simulink model "Two_IBR_Impulse"  (R2022b)
settings: Solver=FixedStepAuto  StartTime=0  StopTime=6  FixedStep=Ts  RelTol=1e-3
undefined symbols (not defined in the file or in its folder): ApparatusDiscreDamping, ApparatusPara, ApparatusPowerFlow, ApparatusType, OtherInputs, R, Ts, Wbase, x_e, Ybase, Zbase
libraries: spsGroundLib x12, SimplusGT x12, spsThreePhaseParallelRLCBranchLib x8, spsThreePhaseBreakerLib x5, spsThreePhaseSeriesRLCBranchLib x3, spspowerguiLib x1
settings Model: Creator=yz34218  LastModifiedBy=yz34218

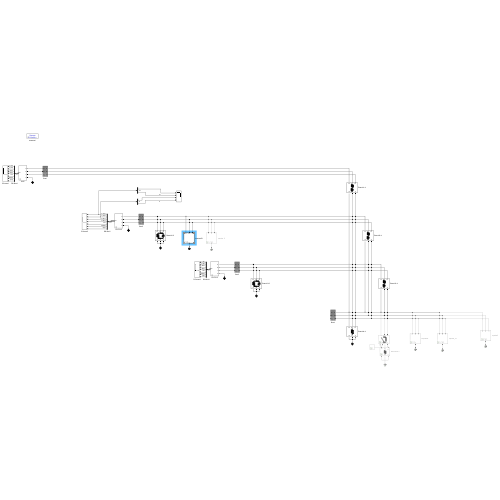
[thumbnail: Simulink's stored preview of the top-level diagram]
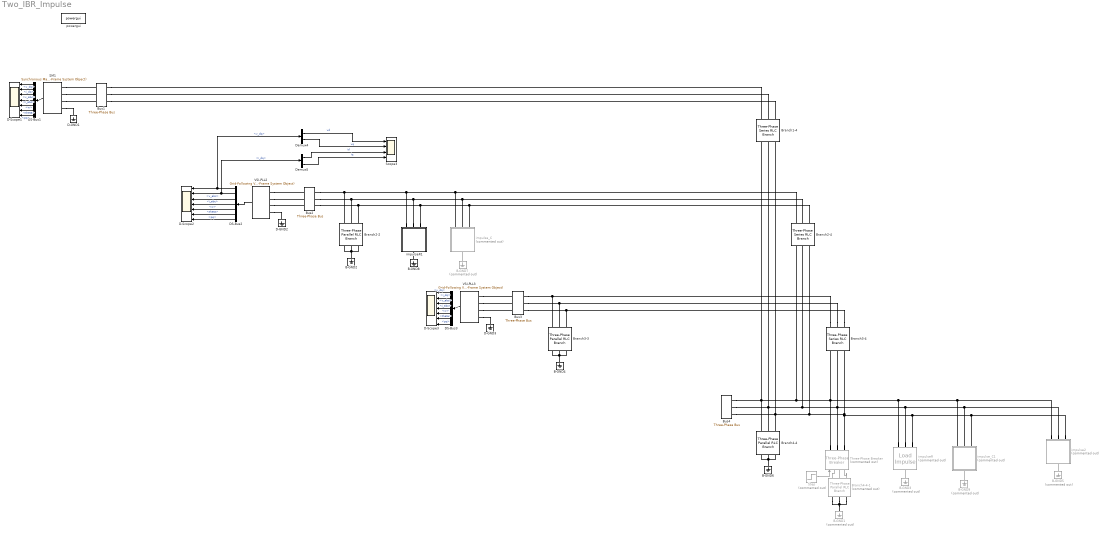
== system Two_IBR_Impulse ==
  B-GND{1,3,5,7,9} (5 alike) : spsGroundLib/Ground  Commented=on  LConnTagsString=a
  B-GND{2,4,6,8} (4 alike) : spsGroundLib/Ground  LConnTagsString=a
  Branch1-4 : spsThreePhaseSeriesRLCBranchLib/Three-Phase Series RLC Branch  LConnTagsString=A|B|C  RConnTagsString=A|B|C  BranchType=RL  Resistance=(0.01)*Zbase  Inductance=(0.1)*Zbase/Wbase  Capacitance=1e-6  Measurements=None
  Branch2-2 : spsThreePhaseParallelRLCBranchLib/Three-Phase Parallel RLC Branch  LConnTagsString=A|B|C  RConnTagsString=A|B|C  BranchType=RC  Resistance=(13.8626)*Zbase  Inductance=(Inf)*Zbase/Wbase  Capacitance=(0.3)*Ybase/Wbase  Measurements=None
  Branch2-4 : spsThreePhaseSeriesRLCBranchLib/Three-Phase Series RLC Branch  LConnTagsString=A|B|C  RConnTagsString=A|B|C  BranchType=RL  Resistance=(0.03)*Zbase  Inductance=(0.3)*Zbase/Wbase  Capacitance=1e-6  Measurements=None
  Branch3-3 : spsThreePhaseParallelRLCBranchLib/Three-Phase Parallel RLC Branch  LConnTagsString=A|B|C  RConnTagsString=A|B|C  BranchType=RC  Resistance=(13.8626)*Zbase  Inductance=(Inf)*Zbase/Wbase  Capacitance=(0.3)*Ybase/Wbase  Measurements=None
  Branch3-4 : spsThreePhaseSeriesRLCBranchLib/Three-Phase Series RLC Branch  LConnTagsString=A|B|C  RConnTagsString=A|B|C  BranchType=RL  Resistance=(0.03)*Zbase  Inductance=(0.3)*Zbase/Wbase  Capacitance=1e-6  Measurements=None
  Branch4-4 : spsThreePhaseParallelRLCBranchLib/Three-Phase Parallel RLC Branch  LConnTagsString=A|B|C  RConnTagsString=A|B|C  BranchType=R  Resistance=(11.3805)*Zbase  Inductance=(Inf)*Zbase/Wbase  Capacitance=(0)*Ybase/Wbase  Measurements=None
  Branch4-4-1 : spsThreePhaseParallelRLCBranchLib/Three-Phase Parallel RLC Branch  Commented=on  LConnTagsString=A|B|C  RConnTagsString=A|B|C  BranchType=R  Resistance=(11.3805)*Zbase*4  Inductance=(Inf)*Zbase/Wbase  Capacitance=(0)*Ybase/Wbase  Measurements=None
  Bus{1..4} (4 alike) : SimplusGT/Three-Phase Bus  Vbase=1  Sbase=1
      settings: SourceProductName=Simplus Grid Tool
  D-GND1 : spsGroundLib/Ground  LConnTagsString=a
  D-GND2 : spsGroundLib/Ground  LConnTagsString=a
  D-GND3 : spsGroundLib/Ground  LConnTagsString=a
  D-Scope1 : Scope  NumInputPorts=7
  D-Scope2 : Scope  NumInputPorts=7
  D-Scope3 : Scope  NumInputPorts=7
  DS-Bus1 : BusSelector  OutputSignals=v_dq,i_dq,v_abc,i_abc,w,theta,pq
  DS-Bus2 : BusSelector  OutputSignals=v_dq,i_dq,v_abc,i_abc,w,theta,pq
  DS-Bus3 : BusSelector  OutputSignals=v_dq,i_dq,v_abc,i_abc,w,theta,pq
  Demux4 : Demux  Outputs=2
  Demux5 : Demux  Outputs=2
  SM1 : SimplusGT/Synchronous Machine (dq-Frame System Object)  Ts=Ts  Sbase=Sbase  Vbase=Vbase  Wbase=Wbase  ApparatusType=ApparatusType{1}  ApparatusPara=ApparatusPara{1}  PowerFlow=ApparatusPowerFlow{1}  x0=x_e{1}  OtherInputs=OtherInputs{1}  DiscreMethod=Hybrid Trapezoidal  EnableInsideModification=off  DiscreDampingFlag=on  DiscreDampingValue=ApparatusDiscreDamping{1}  LinearizationTimes=1  DirectFeedthrough=off
      settings: SourceProductName=Simplus Grid Tool
  Scope3 : Scope  NumInputPorts=4
  Step : Step  Commented=on  Time=3  SampleTime=0
  Three-Phase Breaker : spsThreePhaseBreakerLib/Three-Phase Breaker  Commented=on  InitialState=open  SwitchA=on  SwitchB=on  SwitchC=on  SwitchTimes="[1/60  5/60]"  External=on  BreakerResistance=0.01  SnubberResistance=1e6  SnubberCapacitance=inf  Measurements=None
  VSI-PLL2 : SimplusGT/Grid-Following Voltage-Source Inverter (dq-Frame System Object)  Ts=Ts  Sbase=Sbase  Vbase=Vbase  Wbase=Wbase  ApparatusType=ApparatusType{2}  ApparatusPara=ApparatusPara{2}  PowerFlow=ApparatusPowerFlow{2}  x0=x_e{2}  OtherInputs=OtherInputs{2}  DiscreMethod=Hybrid Trapezoidal  EnableInsideModification=off  DiscreDampingFlag=on  DiscreDampingValue=ApparatusDiscreDamping{2}  LinearizationTimes=1  DirectFeedthrough=off
      settings: SourceProductName=Simplus Grid Tool
  VSI-PLL3 : SimplusGT/Grid-Following Voltage-Source Inverter (dq-Frame System Object)  Ts=Ts  Sbase=Sbase  Vbase=Vbase  Wbase=Wbase  ApparatusType=ApparatusType{3}  ApparatusPara=ApparatusPara{3}  PowerFlow=ApparatusPowerFlow{3}  x0=x_e{3}  OtherInputs=OtherInputs{3}  DiscreMethod=Hybrid Trapezoidal  EnableInsideModification=off  DiscreDampingFlag=on  DiscreDampingValue=ApparatusDiscreDamping{3}  LinearizationTimes=1  DirectFeedthrough=off
      settings: SourceProductName=Simplus Grid Tool
  impulse2 : Subsystem  Commented=on  AncestorBlock=SimplusGT/Load Impulse  mask{t0=6, dt=0.01, C=(11.3805)*Zbase*0.2}
      settings: LibrarySourceBlock=SimplusGT/Load Impulse
  impulseR : SimplusGT/Load Impulse  Commented=on  t0=3  dt=0.01  R=(11.3805)*Zbase*5
      settings: SourceProductName=Simplus Grid Tool
  impulseR1 : Subsystem  AncestorBlock=SimplusGT/Load Impulse  mask{t0=3, dt=0.01, R=(13.8626)*Zbase*2}
      settings: LibrarySourceBlock=SimplusGT/Load Impulse
  impulse_C : Subsystem  Commented=on  AncestorBlock=SimplusGT/Load Impulse  mask{t0=5, dt=0.01, C=(0.3)*Ybase/Wbase*0.1}
      settings: LibrarySourceBlock=SimplusGT/Load Impulse
  impulse_C1 : Subsystem  Commented=on  AncestorBlock=SimplusGT/Load Impulse  mask{t0=6, dt=0.01, C=(0.3)*Ybase/Wbase*0.1}
      settings: LibrarySourceBlock=SimplusGT/Load Impulse
  powergui : spspowerguiLib/powergui  Priority=1  SimulationMode=Discrete  SampleTime=Ts  frequency=60  Iterations=50  frequencyindice=0  Pbase=100e6  ErrMax=1e-4  UnitsV=kV  UnitsW=MW  buscounter=0  FunctionMessages=off  echomessages=off  EnableUseOfTLC=off  CurrentSourceSwitches=off  DisableSnubberDevices=off  DisableRonSwitches=off  DisableVfSwitches=off  DisplayEquations=off  AutomaticDiscreteSolvers=off  SolverType=Tustin/Backward Euler (TBE)  Interpol=off  ExternalGateDelay=off  methode=off  Ts=100  x0status=blocks  SPID=on  SwTol=0  HookPort=off  NonlinearTolerance=1e-4  nMaxIteration=100  ContinueOnMaxIteration=off  RestoreLinks=warning  ResistiveCurrentMeasurement=off  Frange=[0:2:500]  Ylog=off  Xlog=on  ShowGrid=off  save=off  variable=ZData  structure=0  ZoomFFT=off  StartTime=0.0  cycles=1  DisplayStyle=1  fundamental=60  FreqAxis=off  MaxFrequency=1000  frequencyindicesteady=1  RmsSteady=1  display=off
  wires:
  SM1/1 -> DS-Bus1/1
  DS-Bus1/1 -> D-Scope1/1  "<v_dq>"
  DS-Bus1/2 -> D-Scope1/2  "<i_dq>"
  DS-Bus1/3 -> D-Scope1/3  "<v_abc>"
  DS-Bus1/4 -> D-Scope1/4  "<i_abc>"
  DS-Bus1/5 -> D-Scope1/5  "<w>"
  DS-Bus1/6 -> D-Scope1/6  "<theta>"
  DS-Bus1/7 -> D-Scope1/7  "<pq>"
  VSI-PLL2/1 -> DS-Bus2/1
  DS-Bus2/1 -> Demux4/1, D-Scope2/1  "<v_dq>"
  DS-Bus2/2 -> Demux5/1, D-Scope2/2  "<i_dq>"
  DS-Bus2/3 -> D-Scope2/3  "<v_abc>"
  DS-Bus2/4 -> D-Scope2/4  "<i_abc>"
  DS-Bus2/5 -> D-Scope2/5  "<w>"
  DS-Bus2/6 -> D-Scope2/6  "<theta>"
  DS-Bus2/7 -> D-Scope2/7  "<pq>"
  VSI-PLL3/1 -> DS-Bus3/1
  DS-Bus3/2 -> D-Scope3/2  "<i_dq>"
  DS-Bus3/3 -> D-Scope3/3  "<v_abc>"
  DS-Bus3/4 -> D-Scope3/4  "<i_abc>"
  DS-Bus3/5 -> D-Scope3/5  "<w>"
  DS-Bus3/6 -> D-Scope3/6  "<theta>"
  DS-Bus3/7 -> D-Scope3/7  "<pq>"
  Step/1 -> Three-Phase Breaker/1
  DS-Bus3/1 -> D-Scope3/1  "<v_dq>"
  Demux4/2 -> Scope3/2  "vq"
  Demux5/1 -> Scope3/3  "id"
  Demux5/2 -> Scope3/4  "iq"
  Demux4/1 -> Scope3/1  "vd"
  connections:
  SM1/LConn4 -- D-GND1/LConn1
  VSI-PLL2/LConn4 -- D-GND2/LConn1
  VSI-PLL3/LConn4 -- D-GND3/LConn1
  Branch2-2/RConn1 -- Branch2-2/RConn2 -- Branch2-2/RConn3 -- B-GND2/LConn1
  Branch3-3/RConn1 -- Branch3-3/RConn2 -- Branch3-3/RConn3 -- B-GND4/LConn1
  Branch4-4/RConn1 -- Branch4-4/RConn2 -- Branch4-4/RConn3 -- B-GND6/LConn1
  Branch1-4/RConn1 -- Bus4/RConn1 -- Branch4-4/LConn1 -- impulse_C1/LConn1 -- impulse2/LConn1 -- impulseR/LConn1 -- Three-Phase Breaker/RConn1 -- Branch3-4/RConn1 -- Branch2-4/RConn1
  Branch1-4/RConn2 -- Bus4/RConn2 -- Branch4-4/LConn2 -- impulse_C1/LConn2 -- impulse2/LConn2 -- impulseR/LConn2 -- Three-Phase Breaker/RConn2 -- Branch3-4/RConn2 -- Branch2-4/RConn2
  Branch1-4/RConn3 -- Bus4/RConn3 -- Branch4-4/LConn3 -- impulse_C1/LConn3 -- impulse2/LConn3 -- impulseR/LConn3 -- Three-Phase Breaker/RConn3 -- Branch3-4/RConn3 -- Branch2-4/RConn3
  Bus1/RConn1 -- Branch1-4/LConn1
  Bus1/RConn2 -- Branch1-4/LConn2
  Bus1/RConn3 -- Branch1-4/LConn3
  Bus2/RConn1 -- Branch2-2/LConn1 -- Branch2-4/LConn1 -- impulse_C/LConn1 -- impulseR1/LConn1
  Bus2/RConn2 -- Branch2-2/LConn2 -- Branch2-4/LConn2 -- impulse_C/LConn2 -- impulseR1/LConn2
  Bus2/RConn3 -- Branch2-2/LConn3 -- Branch2-4/LConn3 -- impulse_C/LConn3 -- impulseR1/LConn3
  Branch3-4/LConn1 -- Bus3/RConn1 -- Branch3-3/LConn1
  Branch3-4/LConn2 -- Bus3/RConn2 -- Branch3-3/LConn2
  Branch3-4/LConn3 -- Bus3/RConn3 -- Branch3-3/LConn3
  SM1/LConn1 -- Bus1/LConn1
  SM1/LConn2 -- Bus1/LConn2
  SM1/LConn3 -- Bus1/LConn3
  VSI-PLL2/LConn1 -- Bus2/LConn1
  VSI-PLL2/LConn2 -- Bus2/LConn2
  VSI-PLL2/LConn3 -- Bus2/LConn3
  VSI-PLL3/LConn1 -- Bus3/LConn1
  VSI-PLL3/LConn2 -- Bus3/LConn2
  VSI-PLL3/LConn3 -- Bus3/LConn3
  B-GND1/LConn1 -- Branch4-4-1/RConn1 -- Branch4-4-1/RConn3 -- Branch4-4-1/RConn2
  Branch4-4-1/LConn1 -- Three-Phase Breaker/LConn1
  Branch4-4-1/LConn2 -- Three-Phase Breaker/LConn2
  Branch4-4-1/LConn3 -- Three-Phase Breaker/LConn3
  B-GND3/LConn1 -- impulseR/RConn1
  B-GND5/LConn1 -- impulse2/RConn1
  B-GND7/LConn1 -- impulse_C/RConn1
  B-GND8/LConn1 -- impulseR1/RConn1
  B-GND9/LConn1 -- impulse_C1/RConn1

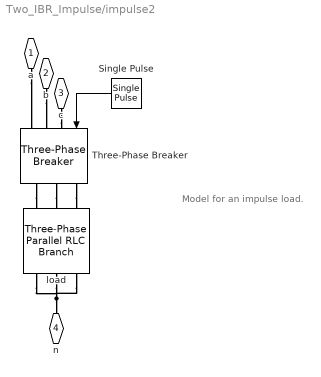
== system Two_IBR_Impulse/impulse2 ==
  note: Model for an impulse load.
  Single Pulse : SimplusGT/Single Pulse  t0=t0  dt=dt  Am=1
      settings: SourceProductName=Simplus Grid Tool
  Three-Phase Breaker : spsThreePhaseBreakerLib/Three-Phase Breaker  InitialState=open  SwitchA=on  SwitchB=on  SwitchC=on  SwitchTimes="[1/60  5/60]"  External=on  BreakerResistance=0.01  SnubberResistance=1e6  SnubberCapacitance=inf  Measurements=None
  load : spsThreePhaseParallelRLCBranchLib/Three-Phase Parallel RLC Branch  LConnTagsString=A|B|C  RConnTagsString=A|B|C  BranchType=C  Resistance=R  Inductance=1  Capacitance=C  Measurements=None
  a : PMIOPort  Side=Left
  b : PMIOPort  Port=2  Side=Left
  c : PMIOPort  Port=3  Side=Left
  n : PMIOPort  Port=4  Side=Right
  wires:
  Single Pulse/1 -> Three-Phase Breaker/1
  connections:
  a/RConn1 -- Three-Phase Breaker/LConn3
  b/RConn1 -- Three-Phase Breaker/LConn2
  c/RConn1 -- Three-Phase Breaker/LConn1
  Three-Phase Breaker/RConn3 -- load/LConn1
  Three-Phase Breaker/RConn2 -- load/LConn2
  Three-Phase Breaker/RConn1 -- load/LConn3
  n/RConn1 -- load/RConn1 -- load/RConn3 -- load/RConn2

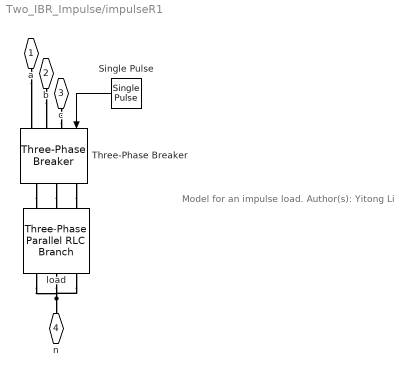
== system Two_IBR_Impulse/impulseR1 ==
  note: Model for an impulse load.
      |
      | Author(s): Yitong Li
  Single Pulse : SimplusGT/Single Pulse  t0=t0  dt=dt  Am=1
      settings: SourceProductName=Simplus Grid Tool
  Three-Phase Breaker : spsThreePhaseBreakerLib/Three-Phase Breaker  InitialState=open  SwitchA=on  SwitchB=on  SwitchC=on  SwitchTimes="[1/60  5/60]"  External=on  BreakerResistance=0.01  SnubberResistance=1e6  SnubberCapacitance=inf  Measurements=None
  load : spsThreePhaseParallelRLCBranchLib/Three-Phase Parallel RLC Branch  LConnTagsString=A|B|C  RConnTagsString=A|B|C  BranchType=R  Resistance=R  Inductance=1  Capacitance=1  Measurements=None
  a : PMIOPort  Side=Left
  b : PMIOPort  Port=2  Side=Left
  c : PMIOPort  Port=3  Side=Left
  n : PMIOPort  Port=4  Side=Right
  wires:
  Single Pulse/1 -> Three-Phase Breaker/1
  connections:
  a/RConn1 -- Three-Phase Breaker/LConn3
  b/RConn1 -- Three-Phase Breaker/LConn2
  c/RConn1 -- Three-Phase Breaker/LConn1
  Three-Phase Breaker/RConn3 -- load/LConn1
  Three-Phase Breaker/RConn2 -- load/LConn2
  Three-Phase Breaker/RConn1 -- load/LConn3
  n/RConn1 -- load/RConn1 -- load/RConn3 -- load/RConn2

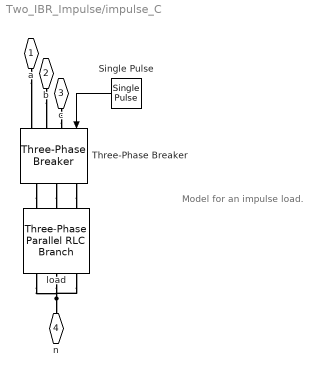
== system Two_IBR_Impulse/impulse_C ==
  note: Model for an impulse load.
  Single Pulse : SimplusGT/Single Pulse  t0=t0  dt=dt  Am=1
      settings: SourceProductName=Simplus Grid Tool
  Three-Phase Breaker : spsThreePhaseBreakerLib/Three-Phase Breaker  InitialState=open  SwitchA=on  SwitchB=on  SwitchC=on  SwitchTimes="[1/60  5/60]"  External=on  BreakerResistance=0.01  SnubberResistance=1e6  SnubberCapacitance=inf  Measurements=None
  load : spsThreePhaseParallelRLCBranchLib/Three-Phase Parallel RLC Branch  LConnTagsString=A|B|C  RConnTagsString=A|B|C  BranchType=C  Resistance=R  Inductance=1  Capacitance=C  Measurements=None
  a : PMIOPort  Side=Left
  b : PMIOPort  Port=2  Side=Left
  c : PMIOPort  Port=3  Side=Left
  n : PMIOPort  Port=4  Side=Right
  wires:
  Single Pulse/1 -> Three-Phase Breaker/1
  connections:
  a/RConn1 -- Three-Phase Breaker/LConn3
  b/RConn1 -- Three-Phase Breaker/LConn2
  c/RConn1 -- Three-Phase Breaker/LConn1
  Three-Phase Breaker/RConn3 -- load/LConn1
  Three-Phase Breaker/RConn2 -- load/LConn2
  Three-Phase Breaker/RConn1 -- load/LConn3
  n/RConn1 -- load/RConn1 -- load/RConn3 -- load/RConn2

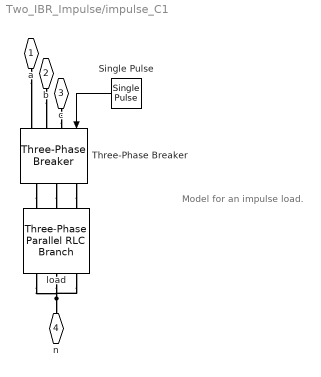
== system Two_IBR_Impulse/impulse_C1 ==
  note: Model for an impulse load.
  Single Pulse : SimplusGT/Single Pulse  t0=t0  dt=dt  Am=1
      settings: SourceProductName=Simplus Grid Tool
  Three-Phase Breaker : spsThreePhaseBreakerLib/Three-Phase Breaker  InitialState=open  SwitchA=on  SwitchB=on  SwitchC=on  SwitchTimes="[1/60  5/60]"  External=on  BreakerResistance=0.01  SnubberResistance=1e6  SnubberCapacitance=inf  Measurements=None
  load : spsThreePhaseParallelRLCBranchLib/Three-Phase Parallel RLC Branch  LConnTagsString=A|B|C  RConnTagsString=A|B|C  BranchType=C  Resistance=R  Inductance=1  Capacitance=C  Measurements=None
  a : PMIOPort  Side=Left
  b : PMIOPort  Port=2  Side=Left
  c : PMIOPort  Port=3  Side=Left
  n : PMIOPort  Port=4  Side=Right
  wires:
  Single Pulse/1 -> Three-Phase Breaker/1
  connections:
  a/RConn1 -- Three-Phase Breaker/LConn3
  b/RConn1 -- Three-Phase Breaker/LConn2
  c/RConn1 -- Three-Phase Breaker/LConn1
  Three-Phase Breaker/RConn3 -- load/LConn1
  Three-Phase Breaker/RConn2 -- load/LConn2
  Three-Phase Breaker/RConn1 -- load/LConn3
  n/RConn1 -- load/RConn1 -- load/RConn3 -- load/RConn2
